simulink model "board_programmer"  (R2021b)
settings: Solver=FixedStepAuto  StartTime=0.0  StopTime=inf  RelTol=1e-3  EnableMultiTasking=on
values from neighbouring files (symbols this model uses):
  circ1 = monza    [board_data.m]
  serial_freq = 50    [board_data.m]
undefined symbols (not defined in the file or in its folder): CR, DiscIntNeverNeededParam, h, LF, pwm, slow, touch
libraries: simulink x19, dspstat3 x14, sharedschedule x12, arduinolib x5, simulink_extras x3, embeddedblockslib x2
settings Model: ExtModeTrigDuration=2  Creator=eduar  LastModifiedBy=ernesto
settings OptimizationCC: EnhancedBackFolding=on  PassReuseOutputArgsAs=Individual arguments  ZeroExternalMemoryAtStartup=off  ZeroInternalMemoryAtStartup=off  MaxStackSize=64  OptimizeBlockOrder=speed  DifferentSizesBufferReuse=on  OptimizationCustomize=off  EfficientTunableParamExpr=on
settings DebuggingCC: ParameterTunabilityLossMsg=error
settings HardwareCC: ProdBitPerPointer=32  ProdBitPerSizeT=32  ProdBitPerPtrDiffT=32  ProdLargestAtomicInteger=Long  ProdLargestAtomicFloat=Double  ProdWordSize=32  ProdHWDeviceType=ARM Compatible->ARM Cortex  UseEmbeddedCoderFeatures=off
settings SFSimCC: SimCustomHeaderCode="#include \"script\\callback.h\""  SimUserSources=script\callback.c  MATLABDynamicMemAlloc=off
settings RTWCC: Description=Embedded Coder  SystemTargetFile=ert.tlc  HardwareBoard=Arduino Due  TemplateMakefile=ert_default_tmf  RTWUseSimCustomCode=on  CustomHeaderCode="#include \"script\\callback.h\""  CustomSource=script\callback.c  Toolchain=Arduino ARM  BuildConfiguration=Faster Runs
settings CodeAppCC: ForceParamTrailComments=on  IgnoreCustomStorageClasses=off  OperatorAnnotations=on  SimulinkDataObjDesc=on  SFDataObjDesc=on  InsertBlockDesc=on
settings ERTTargetCC: SupportContinuousTime=on  SupportNonInlinedSFcns=on  SupportVariableSizeSignals=on  ExtModeTransport=3  ExtModeStaticAlloc=on  ExtModeStaticAllocSize=24576  ExtModeMexFile=ext_xcp  ExtModeIntrfLevel=Level2 - Open

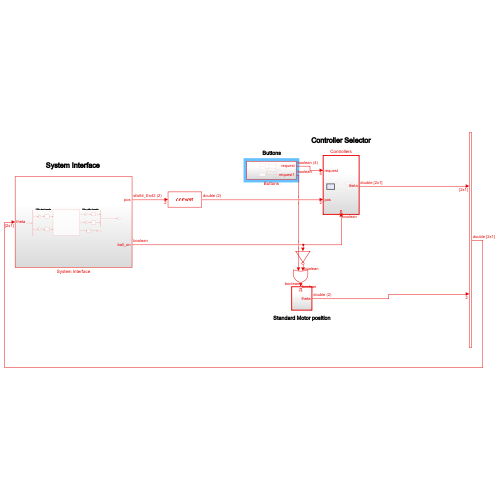
[thumbnail: Simulink's stored preview of the top-level diagram]
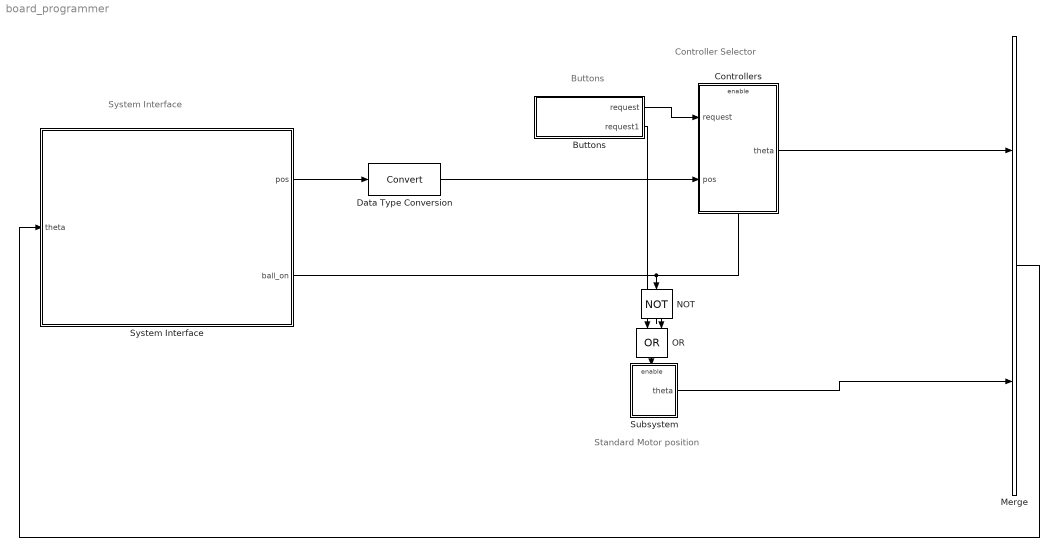
== system board_programmer ==
  note: Standard Motor position
  note: System Interface
  note: Controller Selector
  note: Buttons
  Buttons : Subsystem
  Controllers : Subsystem
  Data Type Conversion : DataTypeConversion
  Merge : Merge
  NOT : Logic  Operator=NOT  IconShape=distinctive  AllPortsSameDT=off  OutDataTypeStr=boolean
  OR : Logic  Operator=OR  IconShape=distinctive  AllPortsSameDT=off  OutDataTypeStr=boolean
  Subsystem : Subsystem
  System Interface : Subsystem
  wires:
  System Interface/1(pos) -> Data Type Conversion/1
  Controllers/1(theta) -> Merge/1
  Merge/1 -> System Interface/1(theta)
  Subsystem/1(theta) -> Merge/2
  System Interface/2(ball_on) -> NOT/1, Controllers/Enable
  Data Type Conversion/1 -> Controllers/2(pos)
  Buttons/1(request) -> Controllers/1(request)
  OR/1 -> Subsystem/Enable
  NOT/1 -> OR/2
  Buttons/2(request1) -> OR/1

== system board_programmer/Buttons ==
  AND : Logic  IconShape=distinctive  AllPortsSameDT=off  OutDataTypeStr=boolean
  Digital Input : arduinolib/Digital Input  pinNumber=7  mode=Input Pullup  Direction=input  SampleTime=0.02  blockPlatform=arduino
  Digital Input1 : arduinolib/Digital Input  pinNumber=53  mode=Input Pullup  Direction=input  SampleTime=0.02  blockPlatform=arduino
  Digital Input2 : arduinolib/Digital Input  pinNumber=51  mode=Input Pullup  Direction=input  SampleTime=0.02  blockPlatform=arduino
  Mux : Mux
  NOT{1..4} (4 alike) : Logic  Operator=NOT  IconShape=distinctive  AllPortsSameDT=off  OutDataTypeStr=boolean
  request : Outport
  request1 : Outport  Port=2
  wires:
  Digital Input1/1 -> AND/1, NOT2/1
  Digital Input2/1 -> AND/2, NOT3/1
  Digital Input/1 -> NOT1/1
  Mux/1 -> request/1
  NOT3/1 -> Mux/4
  AND/1 -> NOT4/1
  NOT4/1 -> request1/1, Mux/3
  NOT2/1 -> Mux/2
  NOT1/1 -> Mux/1

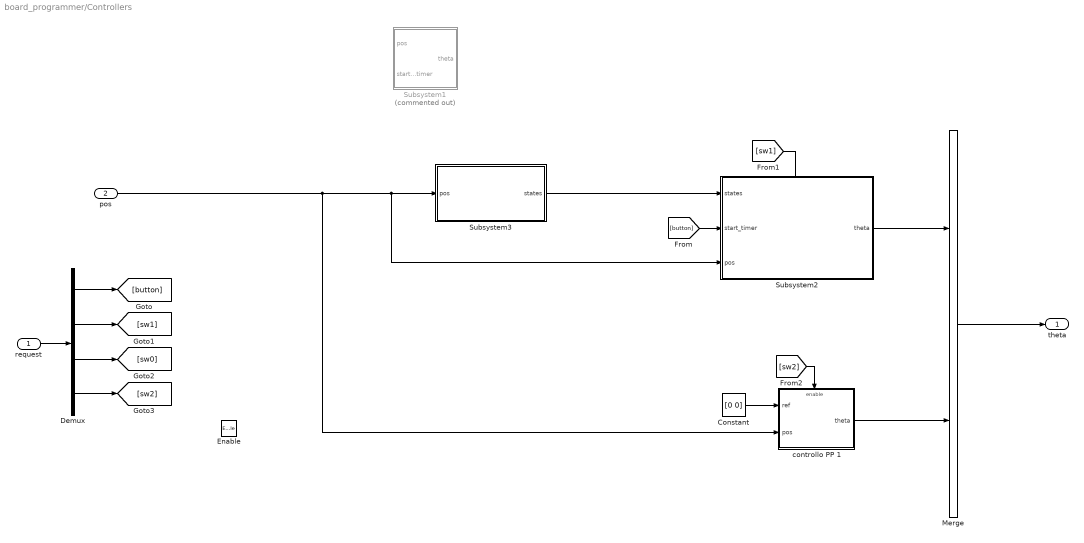
== system board_programmer/Controllers ==
  request : Inport
  pos : Inport  Port=2
  Enable : EnablePort
  Constant : Constant  Value=[0 0]
  Demux : Demux
  Merge : Merge
  Subsystem1 : Subsystem  Commented=on
  Subsystem2 : Subsystem
  Subsystem3 : Subsystem
  controllo PP 1 : Subsystem  SystemSampleTime=0.01
  theta : Outport
  wires:
  Subsystem3/1(states) -> Subsystem2/1(states)
  pos/1 -> controllo PP 1/2("pos "), Subsystem2/3(pos), Subsystem3/1(pos)
  request/1 -> Demux/1
  Demux/1 -> [button]
  Demux/2 -> [sw1]
  Demux/3 -> [sw0]
  Demux/4 -> [sw2]
  [button] -> Subsystem2/2(start_timer)
  [sw1] -> ?
  [sw2] -> controllo PP 1/Enable
  Constant/1 -> controllo PP 1/1("ref ")
  Subsystem2/1(theta) -> Merge/1
  Merge/1 -> theta/1
  controllo PP 1/1(theta) -> Merge/2

== system board_programmer/Subsystem ==
  Enable : EnablePort
  Constant1 : Constant  Value=[0 0]
  theta : Outport
  wires:
  Constant1/1 -> theta/1

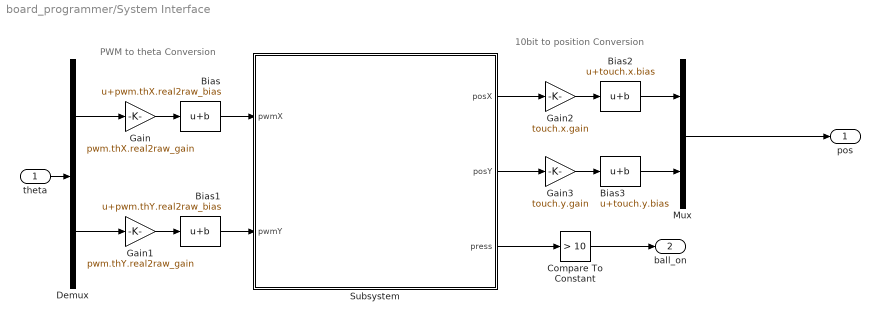
== system board_programmer/System Interface ==
  note: PWM to theta Conversion
  note: 10bit to position Conversion
  theta : Inport
  Bias : Bias  Bias=pwm.thX.real2raw_bias
  Bias1 : Bias  Bias=pwm.thY.real2raw_bias
  Bias2 : Bias  Bias=touch.x.bias
  Bias3 : Bias  Bias=touch.y.bias
  Compare To Constant : simulink/Logic and Bit Operations/Compare To Constant  relop=>  const=10  OutDataTypeStr=boolean
  Demux : Demux  Outputs=2
  Gain : Gain  Gain=pwm.thX.real2raw_gain
  Gain1 : Gain  Gain=pwm.thY.real2raw_gain
  Gain2 : Gain  Gain=touch.x.gain
  Gain3 : Gain  Gain=touch.y.gain
  Mux : Mux  Inputs=2
  Subsystem : Subsystem
  pos : Outport
  ball_on : Outport  Port=2
  wires:
  Subsystem/2(posY) -> Gain3/1
  Subsystem/1(posX) -> Gain2/1
  Bias2/1 -> Mux/1
  Gain/1 -> Bias/1
  Bias/1 -> Subsystem/1(pwmX)
  Demux/1 -> Gain/1
  Mux/1 -> pos/1
  Bias3/1 -> Mux/2
  Bias1/1 -> Subsystem/2(pwmY)
  theta/1 -> Demux/1
  Gain1/1 -> Bias1/1
  Demux/2 -> Gain1/1
  Gain2/1 -> Bias2/1
  Gain3/1 -> Bias3/1
  Subsystem/3(press) -> Compare To Constant/1
  Compare To Constant/1 -> ball_on/1

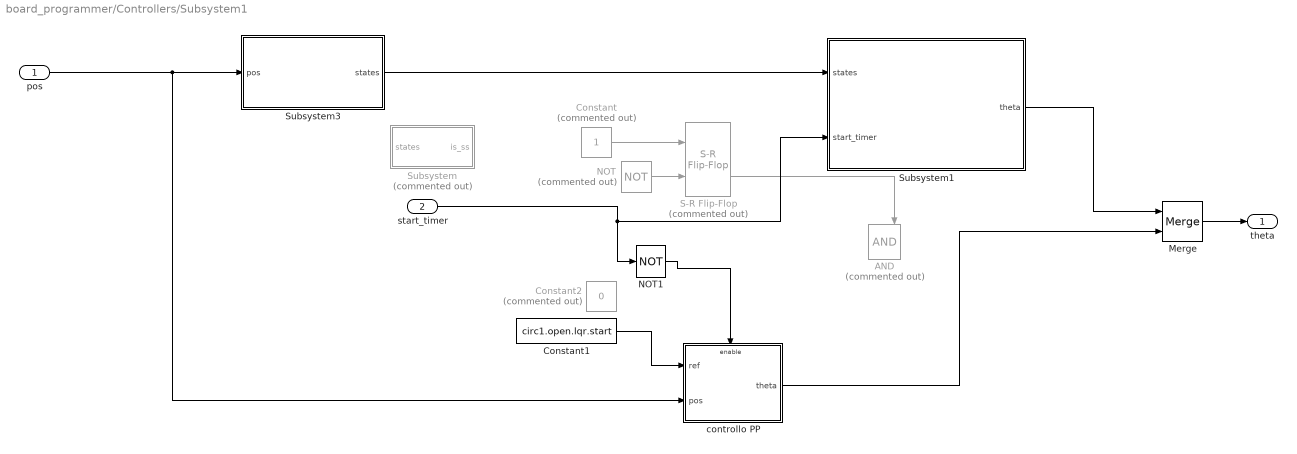
== system board_programmer/Controllers/Subsystem1 ==
  pos : Inport
  start_timer : Inport  Port=2
  AND : Logic  Commented=on  IconShape=distinctive  AllPortsSameDT=off  OutDataTypeStr=boolean
  Constant : Constant  Commented=on  OutDataTypeStr=boolean
  Constant1 : Constant  Value=circ1.open.lqr.start
  Constant2 : Constant  Commented=on  Value=0  OutDataTypeStr=boolean
  Merge : Merge
  NOT : Logic  Commented=on  Operator=NOT  IconShape=distinctive  AllPortsSameDT=off  OutDataTypeStr=boolean
  NOT1 : Logic  Operator=NOT  IconShape=distinctive  AllPortsSameDT=off  OutDataTypeStr=boolean
  S-R Flip-Flop : simulink_extras/Flip Flops/S-R Flip-Flop  Commented=on  initial_condition=0
  Subsystem : Subsystem  Commented=on
  Subsystem1 : Subsystem
  Subsystem3 : Subsystem
  "controllo PP " : Subsystem  SystemSampleTime=0.01
  theta : Outport
  wires:
  Subsystem3/1(states) -> Subsystem1/1(states)
  "controllo PP "/1(theta) -> Merge/2
  pos/1 -> "controllo PP "/2("pos "), Subsystem3/1(pos)
  Constant1/1 -> "controllo PP "/1("ref ")
  NOT/1 -> S-R Flip-Flop/2
  S-R Flip-Flop/2 -> AND/2
  Constant/1 -> S-R Flip-Flop/1
  start_timer/1 -> NOT1/1, Subsystem1/2(start_timer)
  NOT1/1 -> "controllo PP "/Enable
  Subsystem1/1(theta) -> Merge/1
  Merge/1 -> theta/1

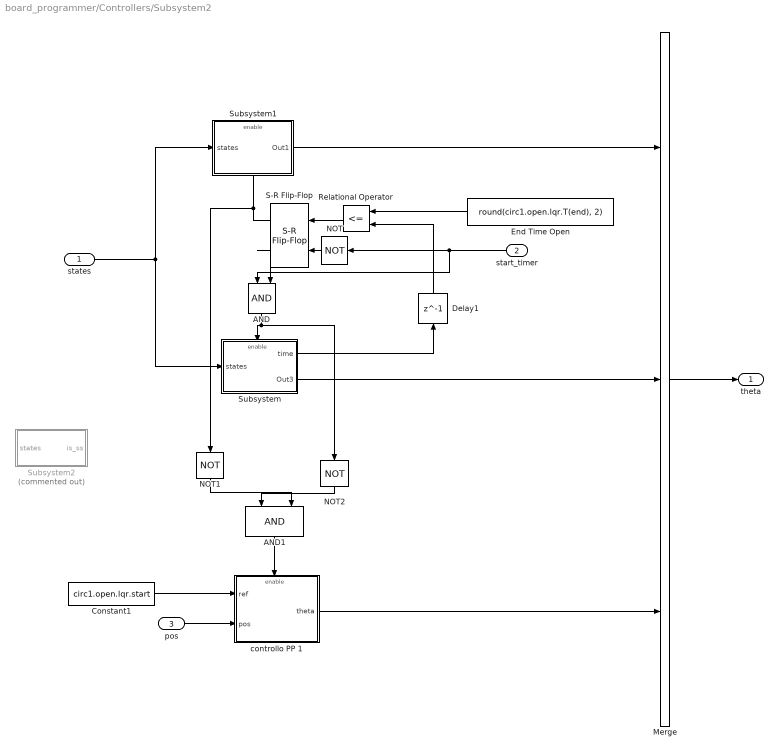
== system board_programmer/Controllers/Subsystem2 ==
  states : Inport
  start_timer : Inport  Port=2
  pos : Inport  Port=3
  AND : Logic  IconShape=distinctive  AllPortsSameDT=off  OutDataTypeStr=boolean
  AND1 : Logic  IconShape=distinctive  AllPortsSameDT=off  OutDataTypeStr=boolean
  Constant1 : Constant  Value=circ1.open.lqr.start
  Delay1 : Delay  DelayLength=1  InitialCondition=0
  End Time Open : Constant  Value=round(circ1.open.lqr.T(end), 2)
  Merge : Merge  Inputs=3
  NOT : Logic  Operator=NOT  IconShape=distinctive  AllPortsSameDT=off  OutDataTypeStr=boolean
  NOT1 : Logic  Operator=NOT  IconShape=distinctive  AllPortsSameDT=off  OutDataTypeStr=boolean
  NOT2 : Logic  Operator=NOT  IconShape=distinctive  AllPortsSameDT=off  OutDataTypeStr=boolean
  Relational Operator : RelationalOperator  Operator=<=  OutDataTypeStr=boolean  RndMeth=Simplest
  S-R Flip-Flop : simulink_extras/Flip Flops/S-R Flip-Flop  initial_condition=0
  Subsystem : Subsystem
  Subsystem1 : Subsystem
  Subsystem2 : Subsystem  Commented=on
  controllo PP 1 : Subsystem  SystemSampleTime=0.01
  theta : Outport
  wires:
  End Time Open/1 -> Relational Operator/1
  Relational Operator/1 -> S-R Flip-Flop/1
  S-R Flip-Flop/2 -> AND/1
  Merge/1 -> theta/1
  states/1 -> Subsystem1/1(states), Subsystem/1(states)
  Subsystem/1(time) -> Delay1/1
  Subsystem/2(Out3) -> Merge/2
  AND/1 -> NOT2/1, Subsystem/Enable
  Subsystem1/1(Out1) -> Merge/1
  S-R Flip-Flop/1 -> NOT1/1, Subsystem1/Enable
  Delay1/1 -> Relational Operator/2
  NOT/1 -> S-R Flip-Flop/2
  Constant1/1 -> controllo PP 1/1("ref ")
  controllo PP 1/1(theta) -> Merge/3
  pos/1 -> controllo PP 1/2("pos ")
  AND1/1 -> controllo PP 1/Enable
  NOT1/1 -> AND1/1
  NOT2/1 -> AND1/2
  start_timer/1 -> AND/2, NOT/1

== system board_programmer/Controllers/Subsystem3 ==
  pos : Inport
  Demux : Demux  Outputs=2
  Discrete Derivative : simulink/Discrete/Discrete Derivative  gainval=1.0  ICPrevScaledInput=0.0  OutMin=[]  OutMax=[]  OutDataType=fixdt(1, 16)  OutScaling=2^-10  DoSatur=off
  Discrete Derivative1 : simulink/Discrete/Discrete Derivative  gainval=1.0  ICPrevScaledInput=0.0  OutMin=[]  OutMax=[]  OutDataType=fixdt(1, 16)  OutScaling=2^-10  DoSatur=off
  Moving Average : dspstat3/Moving Average  Method=Sliding window  ForgettingFactorPort=off  SpecifyWindowLength=on  WindowLength=5  ForgettingFactor=0.9  SimulateUsing=Code generation
  Moving Average1 : dspstat3/Moving Average  Method=Sliding window  ForgettingFactorPort=off  SpecifyWindowLength=on  WindowLength=5  ForgettingFactor=0.9  SimulateUsing=Code generation
  Mux2 : Mux
  states : Outport
  wires:
  Discrete Derivative1/1 -> Moving Average1/1  "Xp [m/s]"
  Mux2/1 -> states/1
  Demux/2 -> Discrete Derivative1/1, Mux2/4
  Discrete Derivative/1 -> Moving Average/1  "Xp [m/s]"
  Demux/1 -> Mux2/2, Discrete Derivative/1
  pos/1 -> Demux/1
  Moving Average/1 -> Mux2/1
  Moving Average1/1 -> Mux2/3

== system board_programmer/Controllers/controllo PP 1 ==
  "ref " : Inport
  "pos " : Inport  Port=2
  Enable : EnablePort  StatesWhenEnabling=reset  ShowOutputPort=on
  Demux : Demux  Outputs=2
  Demux1 : Demux  Outputs=2
  Mux : Mux  Inputs=2
  PPX 1 : Subsystem
  PPX 2 : Subsystem
  Sum2 : Sum  Inputs=|-+
  Sum3 : Sum  Inputs=|-+
  theta : Outport
  wires:
  "ref "/1 -> Demux1/1
  "pos "/1 -> Demux/1
  Demux/1 -> PPX 1/1("pos "), Sum2/1
  Demux/2 -> PPX 2/1("pos "), Sum3/1
  Demux1/1 -> Sum2/2
  Demux1/2 -> Sum3/2
  Sum3/1 -> PPX 2/2(err)
  Sum2/1 -> PPX 1/2(err)
  PPX 2/1(V) -> Mux/2
  PPX 1/1(V) -> Mux/1
  Mux/1 -> theta/1
  Enable/1 -> PPX 2/3(tr), PPX 1/3(tr)

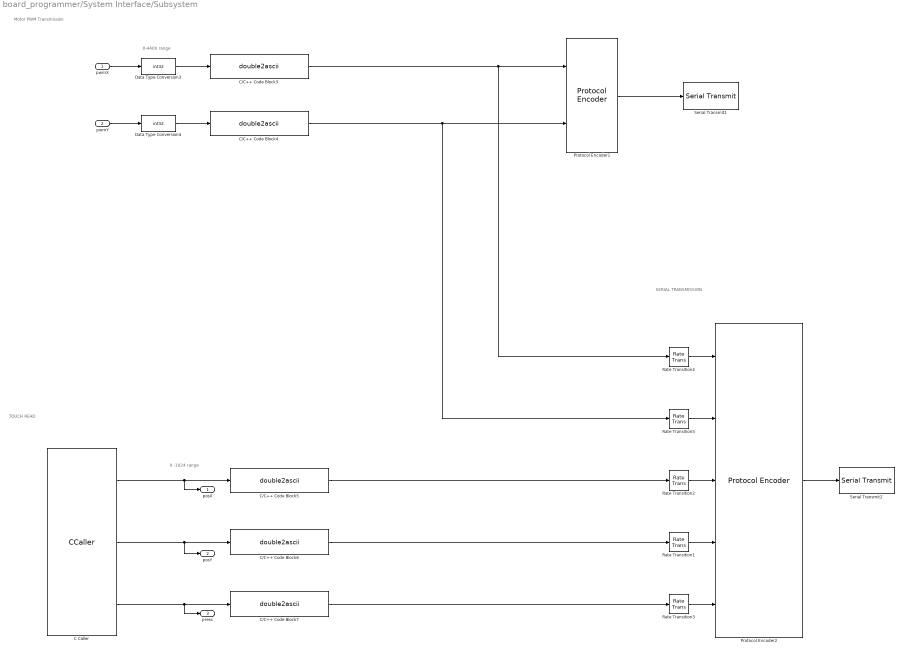
== system board_programmer/System Interface/Subsystem ==
  note: TOUCH READ
  note: Motor PWM Transmission
  note: 0 -1024 range
  note: 0-4400 range
  note: SERIAL TRANSMISSION
  pwmX : Inport
  pwmY : Inport  Port=2
  C Caller : CCaller  FunctionName=touchRead  PortSpecificationStruct="%)30     .    : 4   8    (     @         %    \"     ,    !     0         %  0 \"0    $    _    07)G3F%M90  4&]R=$YA;64 4V-O<&4     26YD97@     5'EP90      4VEZ90      27-';&]B86P   X    P    !@    @    $          4    (     0    $    !         !   0!X    #@   #     &    \"     0         !0    @    !     0    $         $  ! '@    .    .     8    (    !          %    \"     $    &     0         0    !@   $]U='!U=   #@   #@    &    \"     8         !0    @    !     0    $         \"0    @               X    X    !@    @    $          4    (     0    4    !         !     %    :6YT,S(    .    ,     8    (    !          %    \"     $    !     0         0  $ ,0    X    P    !@    @    ) @        4    (     0    $    !          (  0      #@   #     &    \"     0         !0    @    !     0    $         $  ! 'D    .    ,     8    (    !          %    \"     $    !     0         0  $ >0    X    X    !@    @    $          4    (     0    8    !         !     &    3W5T<'5T   .    .     8    (    !@         %    \"     $    !     0         )    \"            / _#@   #@    &    \"     0         !0    @    !    !0    $         $     4   !I;G0S,@    X    P    !@    @    $          4    (     0    $    !         !   0 Q    #@   #     &    \"     D\"        !0    @    !     0    $          @ !       .    .     8    (    !          %    \"     $    %     0         0    !0   '!R97-S    #@   #@    &    \"     0         !0    @    !    !0    $         $     4   !P<F5S<P    X    X    !@    @    $          4    (     0    8    !         !     &    3W5T<'5T   .    .     8    (    !@         %    \"     $    !     0         )    \"             ! #@   #@    &    \"     0         !0    @    !    !0    $         $     4   !I;G0S,@    X    P    !@    @    $          4    (     0    $    !         !   0 Q    #@   #     &    \"     D\"        !0    @    !     0    $          @ !"
  C/C++ Code Block3 : S-Function  FunctionName=double2ascii  SFunctionModules=double2ascii_wrapper  SFunctionDeploymentMode=off  EnableBusSupport=off  mask(S-Function Builder){}
      mask help: Simulink:masks:SFunctionBuilder_MD
      mask init:
      | val = [[.9  0.75 0.75 1 1 .9 .9 1]',[1 1 0.75 0.75 .9 .9 1 .9]'];try , sys = get_param(gcb,'SfunBuilderFcnName');if isempty(sys), sys = get_param(gcb,'FunctionName'); end,catch, sys = get_param(gcb,'FunctionName'); end
      settings: CopyFcn=set_param(gcbh,'LinkStatus','none')  OpenFcn=sfunctionwizard(gcbh)
      mask Display: plot(val(:,1),val(:,2)),disp(sys),port_label('input',1,'double_input'),port_label('output',1,'array_output')
  C/C++ Code Block4 : S-Function  FunctionName=double2ascii  SFunctionModules=double2ascii_wrapper  SFunctionDeploymentMode=off  EnableBusSupport=off  mask(S-Function Builder){}
      mask help: Simulink:masks:SFunctionBuilder_MD
      mask init: same as board_programmer/System Interface/Subsystem/C/C++ Code Block3
      settings: CopyFcn=set_param(gcbh,'LinkStatus','none')  OpenFcn=sfunctionwizard(gcbh)
      mask Display: plot(val(:,1),val(:,2)),disp(sys),port_label('input',1,'double_input'),port_label('output',1,'array_output')
  C/C++ Code Block5 : S-Function  FunctionName=double2ascii  SFunctionModules=double2ascii_wrapper  SFunctionDeploymentMode=off  EnableBusSupport=off  mask(S-Function Builder){}
      mask help: Simulink:masks:SFunctionBuilder_MD
      mask init: same as board_programmer/System Interface/Subsystem/C/C++ Code Block3
      settings: CopyFcn=set_param(gcbh,'LinkStatus','none')  OpenFcn=sfunctionwizard(gcbh)
      mask Display: plot(val(:,1),val(:,2)),disp(sys),port_label('input',1,'double_input'),port_label('output',1,'array_output')
  C/C++ Code Block6 : S-Function  FunctionName=double2ascii  SFunctionModules=double2ascii_wrapper  SFunctionDeploymentMode=off  EnableBusSupport=off  mask(S-Function Builder){}
      mask help: Simulink:masks:SFunctionBuilder_MD
      mask init: same as board_programmer/System Interface/Subsystem/C/C++ Code Block3
      settings: CopyFcn=set_param(gcbh,'LinkStatus','none')  OpenFcn=sfunctionwizard(gcbh)
      mask Display: plot(val(:,1),val(:,2)),disp(sys),port_label('input',1,'double_input'),port_label('output',1,'array_output')
  C/C++ Code Block7 : S-Function  FunctionName=double2ascii  SFunctionModules=double2ascii_wrapper  SFunctionDeploymentMode=off  EnableBusSupport=off  mask(S-Function Builder){}
      mask help: Simulink:masks:SFunctionBuilder_MD
      mask init: same as board_programmer/System Interface/Subsystem/C/C++ Code Block3
      settings: CopyFcn=set_param(gcbh,'LinkStatus','none')  OpenFcn=sfunctionwizard(gcbh)
      mask Display: plot(val(:,1),val(:,2)),disp(sys),port_label('input',1,'double_input'),port_label('output',1,'array_output')
  Data Type Conversion3 : DataTypeConversion  OutDataTypeStr=int32  RndMeth=Round
  Data Type Conversion4 : DataTypeConversion  OutDataTypeStr=int32  RndMeth=Round
  Protocol Encoder1 : embeddedblockslib/Protocol Encoder  Header='@'  FieldTable={ 'motX', '4', 'uint8', 'Little endian'; 'motY ', '4', 'uint8', 'Little endian' }  IsChecksumRequired=off  ChecksumAlgorithm=XOR of bytes  ChecksumSize=[]  TerminatorOption=CR/LF ('\r\n')  CustomTerminatorVal=[]  Logo=ARDUINO
      settings: SourceProductBaseCode=ARDUINO,TIC2000
  Protocol Encoder2 : embeddedblockslib/Protocol Encoder  Header='@'  FieldTable={ 'pwmX', '4', 'uint8', 'Little endian'; 'pwmY', '4', 'uint8', 'Little endian'; 'x', '4', 'uint8', 'Little endian'; 'y', '4', 'uint8', 'Little endian'; 'press', '4', 'uint8', 'Little endian' }  IsChecksumRequired=off  ChecksumAlgorithm=XOR of bytes  ChecksumSize=[]  TerminatorOption=CR/LF ('\r\n')  CustomTerminatorVal=[]  Logo=ARDUINO
      settings: SourceProductBaseCode=ARDUINO,TIC2000
  Rate Transition{1..5} (5 alike) : RateTransition  Integrity=off  OutPortSampleTime=1/serial_freq
  Serial Transmit1 : arduinolib/Serial Transmit  portNumber=3  sendmode=write  sendformat=Decimal  floatprecision=2  blockPlatform=arduino
  Serial Transmit2 : arduinolib/Serial Transmit  portNumber=0  sendmode=write  sendformat=Decimal  floatprecision=2  blockPlatform=arduino
  posX : Outport
  posY : Outport  Port=2
  press : Outport  Port=3
  wires:
  C Caller/2 -> posY/1, C/C++ Code Block6/1
  C/C++ Code Block3/1 -> Rate Transition4/1, Protocol Encoder1/1
  C/C++ Code Block4/1 -> Rate Transition5/1, Protocol Encoder1/2
  C Caller/3 -> press/1, C/C++ Code Block7/1
  C/C++ Code Block7/1 -> Rate Transition3/1
  C Caller/1 -> posX/1, C/C++ Code Block5/1
  C/C++ Code Block6/1 -> Rate Transition1/1
  C/C++ Code Block5/1 -> Rate Transition2/1
  Data Type Conversion4/1 -> C/C++ Code Block4/1
  Protocol Encoder1/1 -> Serial Transmit1/1
  pwmX/1 -> Data Type Conversion3/1
  Data Type Conversion3/1 -> C/C++ Code Block3/1
  pwmY/1 -> Data Type Conversion4/1
  Rate Transition3/1 -> Protocol Encoder2/5
  Rate Transition1/1 -> Protocol Encoder2/4
  Protocol Encoder2/1 -> Serial Transmit2/1
  Rate Transition4/1 -> Protocol Encoder2/1
  Rate Transition5/1 -> Protocol Encoder2/2
  Rate Transition2/1 -> Protocol Encoder2/3

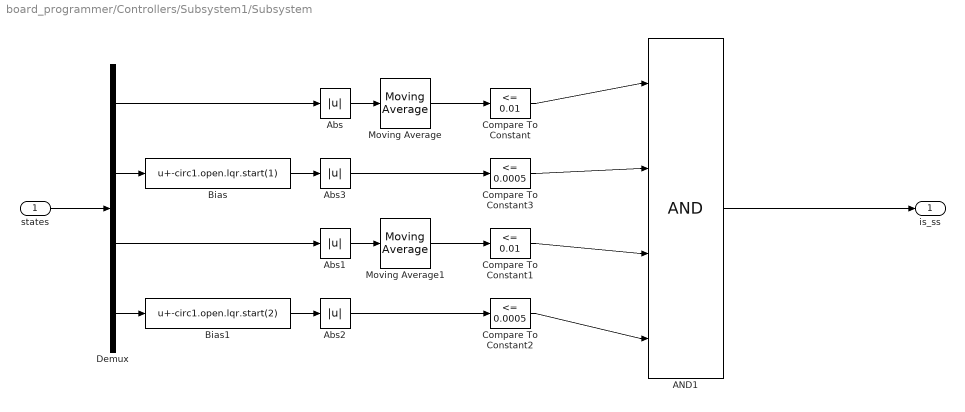
== system board_programmer/Controllers/Subsystem1/Subsystem ==
  states : Inport
  AND1 : Logic  Inputs=4  IconShape=distinctive  AllPortsSameDT=off  OutDataTypeStr=boolean
  Abs{,1..3} (4 alike) : Abs
  Bias : Bias  Bias=-circ1.open.lqr.start(1)
  Bias1 : Bias  Bias=-circ1.open.lqr.start(2)
  Compare To Constant : simulink/Logic and Bit Operations/Compare To Constant  relop=<=  const=0.01  OutDataTypeStr=boolean
  Compare To Constant1 : simulink/Logic and Bit Operations/Compare To Constant  relop=<=  const=0.01  OutDataTypeStr=boolean
  Compare To Constant2 : simulink/Logic and Bit Operations/Compare To Constant  relop=<=  const=0.0005  OutDataTypeStr=boolean
  Compare To Constant3 : simulink/Logic and Bit Operations/Compare To Constant  relop=<=  const=0.0005  OutDataTypeStr=boolean
  Demux : Demux
  Moving Average : dspstat3/Moving Average  Method=Sliding window  ForgettingFactorPort=off  SpecifyWindowLength=on  WindowLength=50  ForgettingFactor=0.9  SimulateUsing=Code generation
  Moving Average1 : dspstat3/Moving Average  Method=Sliding window  ForgettingFactorPort=off  SpecifyWindowLength=on  WindowLength=50  ForgettingFactor=0.9  SimulateUsing=Code generation
  is_ss : Outport
  wires:
  Moving Average1/1 -> Compare To Constant1/1
  Abs1/1 -> Moving Average1/1
  Moving Average/1 -> Compare To Constant/1
  AND1/1 -> is_ss/1
  Abs/1 -> Moving Average/1
  Compare To Constant/1 -> AND1/1
  Demux/1 -> Abs/1
  Demux/3 -> Abs1/1
  Compare To Constant1/1 -> AND1/3
  Demux/2 -> Bias/1
  Demux/4 -> Bias1/1
  Bias1/1 -> Abs2/1
  Bias/1 -> Abs3/1
  Abs2/1 -> Compare To Constant2/1
  Abs3/1 -> Compare To Constant3/1
  Compare To Constant2/1 -> AND1/4
  Compare To Constant3/1 -> AND1/2
  states/1 -> Demux/1

== system board_programmer/Controllers/Subsystem1/Subsystem1 ==
  states : Inport
  start_timer : Inport  Port=2
  AND : Logic  IconShape=distinctive  AllPortsSameDT=off  OutDataTypeStr=boolean
  Delay1 : Delay  DelayLength=1  InitialCondition=0
  End Time Open : Constant  Value=round(circ1.open.lqr.T(end), 2)
  Merge : Merge
  NOT : Logic  Operator=NOT  IconShape=distinctive  AllPortsSameDT=off  OutDataTypeStr=boolean
  Relational Operator : RelationalOperator  Operator=<=  OutDataTypeStr=boolean  RndMeth=Simplest
  S-R Flip-Flop : simulink_extras/Flip Flops/S-R Flip-Flop  initial_condition=0
  Subsystem : Subsystem
  Subsystem1 : Subsystem
  theta : Outport
  wires:
  start_timer/1 -> NOT/1, AND/2
  End Time Open/1 -> Relational Operator/1
  Relational Operator/1 -> S-R Flip-Flop/1
  NOT/1 -> S-R Flip-Flop/2
  S-R Flip-Flop/2 -> AND/1
  Merge/1 -> theta/1
  states/1 -> Subsystem1/1(states), Subsystem/1(states)
  Subsystem/1(time) -> Delay1/1
  Subsystem/2(Out3) -> Merge/2
  AND/1 -> Subsystem/Enable
  Subsystem1/1(Out1) -> Merge/1
  S-R Flip-Flop/1 -> Subsystem1/Enable
  Delay1/1 -> Relational Operator/2

== system board_programmer/Controllers/Subsystem1/Subsystem3 ==
  pos : Inport
  Demux : Demux  Outputs=2
  Discrete Derivative : simulink/Discrete/Discrete Derivative  gainval=1.0  ICPrevScaledInput=0.0  OutMin=[]  OutMax=[]  OutDataType=fixdt(1, 16)  OutScaling=2^-10  DoSatur=off
  Discrete Derivative1 : simulink/Discrete/Discrete Derivative  gainval=1.0  ICPrevScaledInput=0.0  OutMin=[]  OutMax=[]  OutDataType=fixdt(1, 16)  OutScaling=2^-10  DoSatur=off
  Moving Average : dspstat3/Moving Average  Method=Sliding window  ForgettingFactorPort=off  SpecifyWindowLength=on  WindowLength=5  ForgettingFactor=0.9  SimulateUsing=Code generation
  Moving Average1 : dspstat3/Moving Average  Method=Sliding window  ForgettingFactorPort=off  SpecifyWindowLength=on  WindowLength=5  ForgettingFactor=0.9  SimulateUsing=Code generation
  Mux2 : Mux
  states : Outport
  wires:
  Discrete Derivative1/1 -> Moving Average1/1  "Xp [m/s]"
  Mux2/1 -> states/1
  Demux/2 -> Discrete Derivative1/1, Mux2/4
  Discrete Derivative/1 -> Moving Average/1  "Xp [m/s]"
  Demux/1 -> Mux2/2, Discrete Derivative/1
  pos/1 -> Demux/1
  Moving Average/1 -> Mux2/1
  Moving Average1/1 -> Mux2/3

== system board_programmer/Controllers/Subsystem1/controllo PP  ==
  "ref " : Inport
  "pos " : Inport  Port=2
  Enable : EnablePort  StatesWhenEnabling=reset  ShowOutputPort=on
  Demux : Demux  Outputs=2
  Demux1 : Demux  Outputs=2
  Mux : Mux  Inputs=2
  PPX 1 : Subsystem
  PPX 2 : Subsystem
  Sum2 : Sum  Inputs=|-+
  Sum3 : Sum  Inputs=|-+
  theta : Outport
  wires:
  "ref "/1 -> Demux1/1
  "pos "/1 -> Demux/1
  Demux/1 -> PPX 1/1("pos "), Sum2/1
  Demux/2 -> PPX 2/1("pos "), Sum3/1
  Demux1/1 -> Sum2/2
  Demux1/2 -> Sum3/2
  Sum3/1 -> PPX 2/2(err)
  Sum2/1 -> PPX 1/2(err)
  PPX 2/1(V) -> Mux/2
  PPX 1/1(V) -> Mux/1
  Mux/1 -> theta/1
  Enable/1 -> PPX 2/3(tr), PPX 1/3(tr)

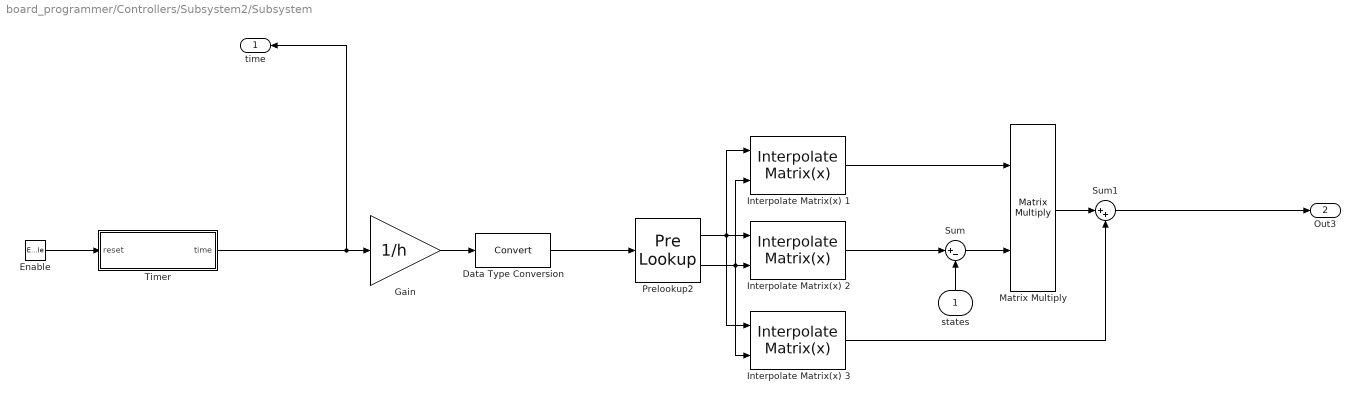
== system board_programmer/Controllers/Subsystem2/Subsystem ==
  states : Inport
  Enable : EnablePort  StatesWhenEnabling=reset  ShowOutputPort=on
  Data Type Conversion : DataTypeConversion
  Gain : Gain  Gain=1/h
  Interpolate Matrix(x) 1 : sharedschedule/Interpolate Matrix(x)   matrix=circ1.open.lqr.K  aMode=aMode
      settings: SourceProductBaseCode=AE,PW,DR,MT,UV,VE
  Interpolate Matrix(x) 2 : sharedschedule/Interpolate Matrix(x)   matrix=circ1.open.lqr.xk  aMode=aMode
      settings: SourceProductBaseCode=AE,PW,DR,MT,UV,VE
  Interpolate Matrix(x) 3 : sharedschedule/Interpolate Matrix(x)   matrix=circ1.open.lqr.uk  aMode=aMode
      settings: SourceProductBaseCode=AE,PW,DR,MT,UV,VE
  Matrix Multiply : Product  Multiplication=Matrix(*)
  Prelookup2 : PreLookup  BreakpointsData=([1:circ1.open.lqr.N])  IndexSearchMethod=Linear search  RemoveProtectionInput=on  BreakpointDataTypeStr=double  FractionDataTypeStr=double
  Sum : Sum  Inputs=|+-
  Sum1 : Sum  Inputs=|++
  "Timer " : Subsystem  TreatAsAtomicUnit=on
  time : Outport
  Out3 : Outport  Port=2
  wires:
  Interpolate Matrix(x) 2/1 -> Sum/1
  Data Type Conversion/1 -> Prelookup2/1
  Matrix Multiply/1 -> Sum1/1
  Interpolate Matrix(x) 3/1 -> Sum1/2
  Prelookup2/1 -> Interpolate Matrix(x) 1/1, Interpolate Matrix(x) 3/1, Interpolate Matrix(x) 2/1
  states/1 -> Sum/2
  Sum/1 -> Matrix Multiply/2
  "Timer "/1(time) -> time/1, Gain/1
  Gain/1 -> Data Type Conversion/1
  Prelookup2/2 -> Interpolate Matrix(x) 3/2, Interpolate Matrix(x) 1/2, Interpolate Matrix(x) 2/2
  Interpolate Matrix(x) 1/1 -> Matrix Multiply/1
  Sum1/1 -> Out3/1
  Enable/1 -> "Timer "/1(reset)

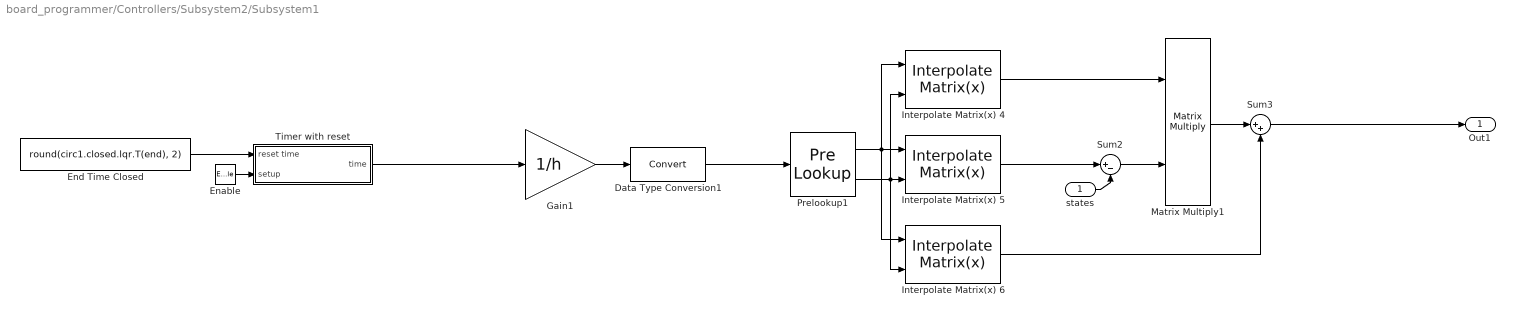
== system board_programmer/Controllers/Subsystem2/Subsystem1 ==
  states : Inport
  Enable : EnablePort  StatesWhenEnabling=reset  ShowOutputPort=on
  Data Type Conversion1 : DataTypeConversion
  End Time Closed : Constant  Value=round(circ1.closed.lqr.T(end), 2)
  Gain1 : Gain  Gain=1/h
  Interpolate Matrix(x) 4 : sharedschedule/Interpolate Matrix(x)   matrix=circ1.open.lqr.K  aMode=aMode
      settings: SourceProductBaseCode=AE,PW,DR,MT,UV,VE
  Interpolate Matrix(x) 5 : sharedschedule/Interpolate Matrix(x)   matrix=circ1.open.lqr.xk  aMode=aMode
      settings: SourceProductBaseCode=AE,PW,DR,MT,UV,VE
  Interpolate Matrix(x) 6 : sharedschedule/Interpolate Matrix(x)   matrix=circ1.open.lqr.uk  aMode=aMode
      settings: SourceProductBaseCode=AE,PW,DR,MT,UV,VE
  Matrix Multiply1 : Product  Multiplication=Matrix(*)
  Prelookup1 : PreLookup  BreakpointsData=([1:circ1.open.lqr.N])  IndexSearchMethod=Linear search  RemoveProtectionInput=on  BreakpointDataTypeStr=double  FractionDataTypeStr=double
  Sum2 : Sum  Inputs=|+-
  Sum3 : Sum  Inputs=|++
  Timer with reset : Subsystem  TreatAsAtomicUnit=on
  Out1 : Outport
  wires:
  Prelookup1/2 -> Interpolate Matrix(x) 6/2, Interpolate Matrix(x) 4/2, Interpolate Matrix(x) 5/2
  Prelookup1/1 -> Interpolate Matrix(x) 4/1, Interpolate Matrix(x) 6/1, Interpolate Matrix(x) 5/1
  Data Type Conversion1/1 -> Prelookup1/1
  Sum2/1 -> Matrix Multiply1/2
  Interpolate Matrix(x) 6/1 -> Sum3/2
  Gain1/1 -> Data Type Conversion1/1
  Interpolate Matrix(x) 5/1 -> Sum2/1
  Matrix Multiply1/1 -> Sum3/1
  End Time Closed/1 -> Timer with reset/1(reset time)
  Interpolate Matrix(x) 4/1 -> Matrix Multiply1/1
  Timer with reset/1(time) -> Gain1/1
  Sum3/1 -> Out1/1
  states/1 -> Sum2/2
  Enable/1 -> Timer with reset/2(setup)

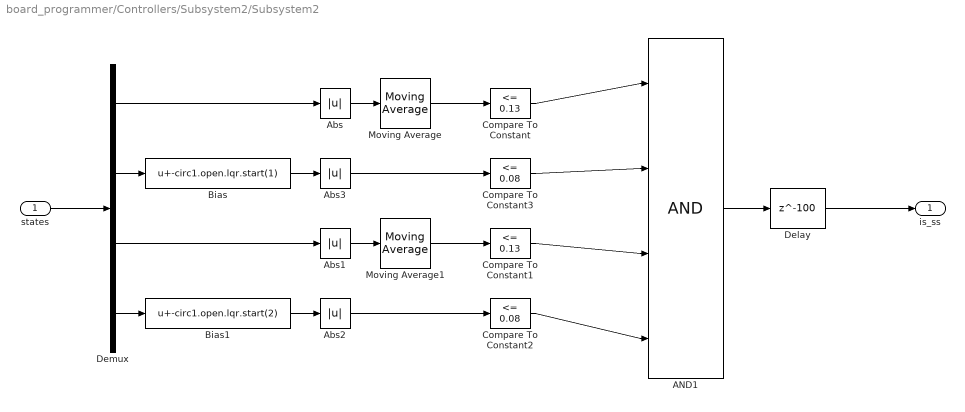
== system board_programmer/Controllers/Subsystem2/Subsystem2 ==
  states : Inport
  AND1 : Logic  Inputs=4  IconShape=distinctive  AllPortsSameDT=off  OutDataTypeStr=boolean
  Abs{,1..3} (4 alike) : Abs
  Bias : Bias  Bias=-circ1.open.lqr.start(1)
  Bias1 : Bias  Bias=-circ1.open.lqr.start(2)
  Compare To Constant : simulink/Logic and Bit Operations/Compare To Constant  relop=<=  const=0.13  OutDataTypeStr=boolean
  Compare To Constant1 : simulink/Logic and Bit Operations/Compare To Constant  relop=<=  const=0.13  OutDataTypeStr=boolean
  Compare To Constant2 : simulink/Logic and Bit Operations/Compare To Constant  relop=<=  const=0.08  OutDataTypeStr=boolean
  Compare To Constant3 : simulink/Logic and Bit Operations/Compare To Constant  relop=<=  const=0.08  OutDataTypeStr=boolean
  Delay : Delay  DelayLength=100  InputProcessing=Columns as channels (frame based)
  Demux : Demux
  Moving Average : dspstat3/Moving Average  Method=Sliding window  ForgettingFactorPort=off  SpecifyWindowLength=on  WindowLength=50  ForgettingFactor=0.9  SimulateUsing=Code generation
  Moving Average1 : dspstat3/Moving Average  Method=Sliding window  ForgettingFactorPort=off  SpecifyWindowLength=on  WindowLength=50  ForgettingFactor=0.9  SimulateUsing=Code generation
  is_ss : Outport
  wires:
  Moving Average1/1 -> Compare To Constant1/1
  Abs1/1 -> Moving Average1/1
  Moving Average/1 -> Compare To Constant/1
  AND1/1 -> Delay/1
  Abs/1 -> Moving Average/1
  Compare To Constant/1 -> AND1/1
  Demux/1 -> Abs/1
  Demux/3 -> Abs1/1
  Compare To Constant1/1 -> AND1/3
  Demux/2 -> Bias/1
  Demux/4 -> Bias1/1
  Bias1/1 -> Abs2/1
  Bias/1 -> Abs3/1
  Abs2/1 -> Compare To Constant2/1
  Abs3/1 -> Compare To Constant3/1
  Compare To Constant2/1 -> AND1/4
  Compare To Constant3/1 -> AND1/2
  states/1 -> Demux/1
  Delay/1 -> is_ss/1

== system board_programmer/Controllers/Subsystem2/controllo PP 1 ==
  "ref " : Inport
  "pos " : Inport  Port=2
  Enable : EnablePort  StatesWhenEnabling=reset  ShowOutputPort=on
  Demux : Demux  Outputs=2
  Demux1 : Demux  Outputs=2
  Mux : Mux  Inputs=2
  PPX 1 : Subsystem
  PPX 2 : Subsystem
  Sum2 : Sum  Inputs=|-+
  Sum3 : Sum  Inputs=|-+
  theta : Outport
  wires:
  "ref "/1 -> Demux1/1
  "pos "/1 -> Demux/1
  Demux/1 -> PPX 1/1("pos "), Sum2/1
  Demux/2 -> PPX 2/1("pos "), Sum3/1
  Demux1/1 -> Sum2/2
  Demux1/2 -> Sum3/2
  Sum3/1 -> PPX 2/2(err)
  Sum2/1 -> PPX 1/2(err)
  PPX 2/1(V) -> Mux/2
  PPX 1/1(V) -> Mux/1
  Mux/1 -> theta/1
  Enable/1 -> PPX 2/3(tr), PPX 1/3(tr)

== system board_programmer/Controllers/controllo PP 1/PPX 1 ==
  note: theta_x
  note: x_vel
  "pos " : Inport
  err : Inport  Port=2
  tr : Inport  Port=3
  Delay : Delay  DelayLength=1  InitialCondition=0
  Discrete Derivative : simulink/Discrete/Discrete Derivative  gainval=1.0  ICPrevScaledInput=0.0  OutMin=[]  OutMax=[]  OutDataType=fixdt(1, 16)  OutScaling=2^-10  DoSatur=off
  Discrete-Time Integrator : DiscreteIntegrator  ExternalReset=rising  SampleTime=-1  ICPrevOutput=DiscIntNeverNeededParam  ICPrevScaledInput=DiscIntNeverNeededParam
  Moving Average : dspstat3/Moving Average  Method=Sliding window  ForgettingFactorPort=off  SpecifyWindowLength=on  WindowLength=10  ForgettingFactor=0.9  SimulateUsing=Code generation
  Mux1 : Mux  Inputs=3
  Sum1 : Sum  Inputs=+|+
  Unary Minus : UnaryMinus
  x integration gain : Gain  Gain=slow.Kxi  Multiplication=Matrix(K*u)
  x matrix gain : Gain  Gain=slow.Kx  Multiplication=Matrix(K*u)
  V : Outport
  wires:
  x matrix gain/1 -> Sum1/1
  Mux1/1 -> x matrix gain/1  "x_vector"
  x integration gain/1 -> Sum1/2
  err/1 -> Discrete-Time Integrator/1, Mux1/2  "x_pos"
  Discrete-Time Integrator/1 -> x integration gain/1  "int_x"
  "pos "/1 -> Discrete Derivative/1
  Delay/1 -> Mux1/3
  Sum1/1 -> Delay/1, V/1
  tr/1 -> Discrete-Time Integrator/2  "x_pos"
  Discrete Derivative/1 -> Unary Minus/1
  Unary Minus/1 -> Moving Average/1
  Moving Average/1 -> Mux1/1

== system board_programmer/Controllers/controllo PP 1/PPX 2 ==
  note: theta_x
  note: x_vel
  "pos " : Inport
  err : Inport  Port=2
  tr : Inport  Port=3
  Delay : Delay  DelayLength=1  InitialCondition=0
  Discrete Derivative : simulink/Discrete/Discrete Derivative  gainval=1.0  ICPrevScaledInput=0.0  OutMin=[]  OutMax=[]  OutDataType=fixdt(1, 16)  OutScaling=2^-10  DoSatur=off
  Discrete-Time Integrator : DiscreteIntegrator  ExternalReset=rising  SampleTime=-1  ICPrevOutput=DiscIntNeverNeededParam  ICPrevScaledInput=DiscIntNeverNeededParam
  Moving Average : dspstat3/Moving Average  Method=Sliding window  ForgettingFactorPort=off  SpecifyWindowLength=on  WindowLength=10  ForgettingFactor=0.9  SimulateUsing=Code generation
  Mux1 : Mux  Inputs=3
  Sum1 : Sum  Inputs=+|+
  Unary Minus : UnaryMinus
  x integration gain : Gain  Gain=slow.Kyi  Multiplication=Matrix(K*u)
  x matrix gain : Gain  Gain=slow.Ky  Multiplication=Matrix(K*u)
  V : Outport
  wires:
  x matrix gain/1 -> Sum1/1
  Mux1/1 -> x matrix gain/1  "x_vector"
  x integration gain/1 -> Sum1/2
  err/1 -> Discrete-Time Integrator/1, Mux1/2  "x_pos"
  Discrete-Time Integrator/1 -> x integration gain/1  "int_x"
  "pos "/1 -> Discrete Derivative/1
  Delay/1 -> Mux1/3
  Sum1/1 -> Delay/1, V/1
  tr/1 -> Discrete-Time Integrator/2  "x_pos"
  Discrete Derivative/1 -> Unary Minus/1
  Unary Minus/1 -> Moving Average/1
  Moving Average/1 -> Mux1/1

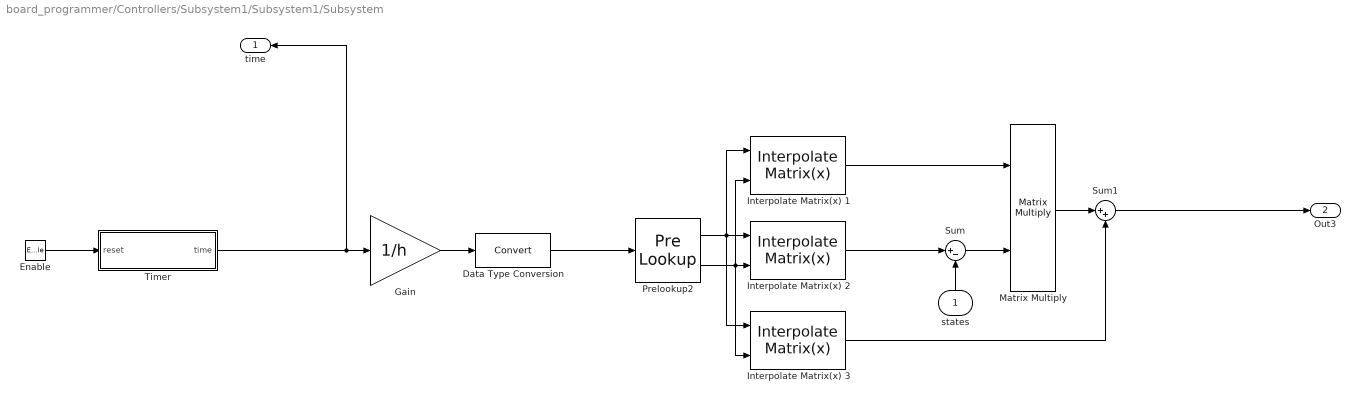
== system board_programmer/Controllers/Subsystem1/Subsystem1/Subsystem ==
  states : Inport
  Enable : EnablePort  StatesWhenEnabling=reset  ShowOutputPort=on
  Data Type Conversion : DataTypeConversion
  Gain : Gain  Gain=1/h
  Interpolate Matrix(x) 1 : sharedschedule/Interpolate Matrix(x)   matrix=circ1.open.lqr.K  aMode=aMode
      settings: SourceProductBaseCode=AE,PW,DR,MT,UV,VE
  Interpolate Matrix(x) 2 : sharedschedule/Interpolate Matrix(x)   matrix=circ1.open.lqr.xk  aMode=aMode
      settings: SourceProductBaseCode=AE,PW,DR,MT,UV,VE
  Interpolate Matrix(x) 3 : sharedschedule/Interpolate Matrix(x)   matrix=circ1.open.lqr.uk  aMode=aMode
      settings: SourceProductBaseCode=AE,PW,DR,MT,UV,VE
  Matrix Multiply : Product  Multiplication=Matrix(*)
  Prelookup2 : PreLookup  BreakpointsData=([1:circ1.open.lqr.N])  IndexSearchMethod=Linear search  RemoveProtectionInput=on  BreakpointDataTypeStr=double  FractionDataTypeStr=double
  Sum : Sum  Inputs=|+-
  Sum1 : Sum  Inputs=|++
  "Timer " : Subsystem  TreatAsAtomicUnit=on
  time : Outport
  Out3 : Outport  Port=2
  wires:
  Interpolate Matrix(x) 2/1 -> Sum/1
  Data Type Conversion/1 -> Prelookup2/1
  Matrix Multiply/1 -> Sum1/1
  Interpolate Matrix(x) 3/1 -> Sum1/2
  Prelookup2/1 -> Interpolate Matrix(x) 1/1, Interpolate Matrix(x) 3/1, Interpolate Matrix(x) 2/1
  states/1 -> Sum/2
  Sum/1 -> Matrix Multiply/2
  "Timer "/1(time) -> time/1, Gain/1
  Gain/1 -> Data Type Conversion/1
  Prelookup2/2 -> Interpolate Matrix(x) 3/2, Interpolate Matrix(x) 1/2, Interpolate Matrix(x) 2/2
  Interpolate Matrix(x) 1/1 -> Matrix Multiply/1
  Sum1/1 -> Out3/1
  Enable/1 -> "Timer "/1(reset)

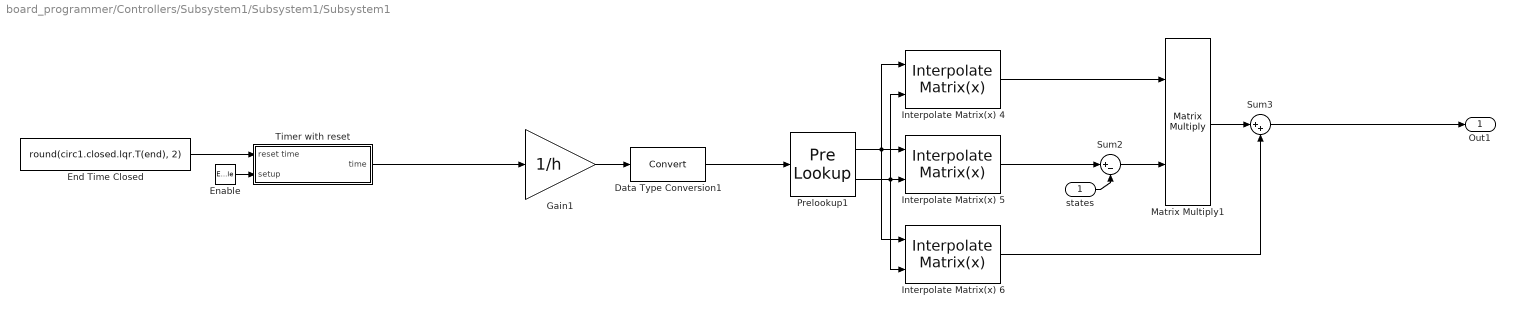
== system board_programmer/Controllers/Subsystem1/Subsystem1/Subsystem1 ==
  states : Inport
  Enable : EnablePort  StatesWhenEnabling=reset  ShowOutputPort=on
  Data Type Conversion1 : DataTypeConversion
  End Time Closed : Constant  Value=round(circ1.closed.lqr.T(end), 2)
  Gain1 : Gain  Gain=1/h
  Interpolate Matrix(x) 4 : sharedschedule/Interpolate Matrix(x)   matrix=circ1.open.lqr.K  aMode=aMode
      settings: SourceProductBaseCode=AE,PW,DR,MT,UV,VE
  Interpolate Matrix(x) 5 : sharedschedule/Interpolate Matrix(x)   matrix=circ1.open.lqr.xk  aMode=aMode
      settings: SourceProductBaseCode=AE,PW,DR,MT,UV,VE
  Interpolate Matrix(x) 6 : sharedschedule/Interpolate Matrix(x)   matrix=circ1.open.lqr.uk  aMode=aMode
      settings: SourceProductBaseCode=AE,PW,DR,MT,UV,VE
  Matrix Multiply1 : Product  Multiplication=Matrix(*)
  Prelookup1 : PreLookup  BreakpointsData=([1:circ1.open.lqr.N])  IndexSearchMethod=Linear search  RemoveProtectionInput=on  BreakpointDataTypeStr=double  FractionDataTypeStr=double
  Sum2 : Sum  Inputs=|+-
  Sum3 : Sum  Inputs=|++
  Timer with reset : Subsystem  TreatAsAtomicUnit=on
  Out1 : Outport
  wires:
  Prelookup1/2 -> Interpolate Matrix(x) 6/2, Interpolate Matrix(x) 4/2, Interpolate Matrix(x) 5/2
  Prelookup1/1 -> Interpolate Matrix(x) 4/1, Interpolate Matrix(x) 6/1, Interpolate Matrix(x) 5/1
  Data Type Conversion1/1 -> Prelookup1/1
  Sum2/1 -> Matrix Multiply1/2
  Interpolate Matrix(x) 6/1 -> Sum3/2
  Gain1/1 -> Data Type Conversion1/1
  Interpolate Matrix(x) 5/1 -> Sum2/1
  Matrix Multiply1/1 -> Sum3/1
  End Time Closed/1 -> Timer with reset/1(reset time)
  Interpolate Matrix(x) 4/1 -> Matrix Multiply1/1
  Timer with reset/1(time) -> Gain1/1
  Sum3/1 -> Out1/1
  states/1 -> Sum2/2
  Enable/1 -> Timer with reset/2(setup)

== system board_programmer/Controllers/Subsystem1/controllo PP /PPX 1 ==
  note: theta_x
  note: x_vel
  "pos " : Inport
  err : Inport  Port=2
  tr : Inport  Port=3
  Delay : Delay  DelayLength=1  InitialCondition=0
  Discrete Derivative : simulink/Discrete/Discrete Derivative  gainval=1.0  ICPrevScaledInput=0.0  OutMin=[]  OutMax=[]  OutDataType=fixdt(1, 16)  OutScaling=2^-10  DoSatur=off
  Discrete-Time Integrator : DiscreteIntegrator  ExternalReset=rising  SampleTime=-1  ICPrevOutput=DiscIntNeverNeededParam  ICPrevScaledInput=DiscIntNeverNeededParam
  Gain : Gain  Gain=0.15
  Moving Average : dspstat3/Moving Average  Method=Sliding window  ForgettingFactorPort=off  SpecifyWindowLength=on  WindowLength=20  ForgettingFactor=0.9  SimulateUsing=Code generation
  Mux1 : Mux  Inputs=3
  Sum1 : Sum  Inputs=+|+
  Unary Minus : UnaryMinus
  x integration gain : Gain  Gain=slow.Kxi  Multiplication=Matrix(K*u)
  x matrix gain : Gain  Gain=slow.Kx  Multiplication=Matrix(K*u)
  V : Outport
  wires:
  x matrix gain/1 -> Sum1/1
  Mux1/1 -> x matrix gain/1  "x_vector"
  x integration gain/1 -> Sum1/2
  err/1 -> Discrete-Time Integrator/1, Mux1/2  "x_pos"
  Discrete-Time Integrator/1 -> x integration gain/1  "int_x"
  Sum1/1 -> Gain/1
  "pos "/1 -> Discrete Derivative/1
  Delay/1 -> Mux1/3
  Gain/1 -> Delay/1, V/1
  tr/1 -> Discrete-Time Integrator/2  "x_pos"
  Discrete Derivative/1 -> Unary Minus/1
  Unary Minus/1 -> Moving Average/1
  Moving Average/1 -> Mux1/1

== system board_programmer/Controllers/Subsystem1/controllo PP /PPX 2 ==
  note: theta_x
  note: x_vel
  "pos " : Inport
  err : Inport  Port=2
  tr : Inport  Port=3
  Delay : Delay  DelayLength=1  InitialCondition=0
  Discrete Derivative : simulink/Discrete/Discrete Derivative  gainval=1.0  ICPrevScaledInput=0.0  OutMin=[]  OutMax=[]  OutDataType=fixdt(1, 16)  OutScaling=2^-10  DoSatur=off
  Discrete-Time Integrator : DiscreteIntegrator  ExternalReset=rising  SampleTime=-1  ICPrevOutput=DiscIntNeverNeededParam  ICPrevScaledInput=DiscIntNeverNeededParam
  Gain : Gain  Gain=0.15
  Moving Average : dspstat3/Moving Average  Method=Sliding window  ForgettingFactorPort=off  SpecifyWindowLength=on  WindowLength=10  ForgettingFactor=0.9  SimulateUsing=Code generation
  Mux1 : Mux  Inputs=3
  Sum1 : Sum  Inputs=+|+
  x integration gain : Gain  Gain=slow.Kyi  Multiplication=Matrix(K*u)
  x matrix gain : Gain  Gain=slow.Ky  Multiplication=Matrix(K*u)
  V : Outport
  wires:
  x matrix gain/1 -> Sum1/1
  Mux1/1 -> x matrix gain/1  "x_vector"
  x integration gain/1 -> Sum1/2
  err/1 -> Discrete-Time Integrator/1, Mux1/2  "x_pos"
  Discrete-Time Integrator/1 -> x integration gain/1  "int_x"
  Sum1/1 -> Gain/1
  "pos "/1 -> Discrete Derivative/1
  Delay/1 -> Mux1/3
  Gain/1 -> Delay/1, V/1
  tr/1 -> Discrete-Time Integrator/2  "x_pos"
  Discrete Derivative/1 -> Moving Average/1
  Moving Average/1 -> Mux1/1

== system board_programmer/Controllers/Subsystem2/Subsystem/Timer  ==
  reset : Inport
  Constant : Constant  SampleTime=-1
  Discrete-Time Integrator : DiscreteIntegrator  ExternalReset=either  SampleTime=-1  ICPrevOutput=DiscIntNeverNeededParam  ICPrevScaledInput=DiscIntNeverNeededParam
  time : Outport
  wires:
  Constant/1 -> Discrete-Time Integrator/1
  Discrete-Time Integrator/1 -> time/1
  reset/1 -> Discrete-Time Integrator/2

== system board_programmer/Controllers/Subsystem2/Subsystem1/Timer with reset ==
  reset time : Inport
  setup : Inport  Port=2
  AND : Logic  IconShape=distinctive  AllPortsSameDT=off  OutDataTypeStr=boolean
  Constant : Constant  SampleTime=-1
  Delay1 : Delay  DelayLength=1  InitialCondition=0
  Discrete-Time Integrator : DiscreteIntegrator  ExternalReset=either  SampleTime=-1  ICPrevOutput=DiscIntNeverNeededParam  ICPrevScaledInput=DiscIntNeverNeededParam
  Relational Operator : RelationalOperator  OutDataTypeStr=boolean  RndMeth=Simplest
  time : Outport
  wires:
  Constant/1 -> Discrete-Time Integrator/1
  Discrete-Time Integrator/1 -> Delay1/1, time/1
  AND/1 -> Discrete-Time Integrator/2
  setup/1 -> AND/1
  reset time/1 -> Relational Operator/2
  Delay1/1 -> Relational Operator/1
  Relational Operator/1 -> AND/2

== system board_programmer/Controllers/Subsystem2/controllo PP 1/PPX 1 ==
  note: theta_x
  note: x_vel
  "pos " : Inport
  err : Inport  Port=2
  tr : Inport  Port=3
  Delay : Delay  DelayLength=1  InitialCondition=0
  Discrete Derivative : simulink/Discrete/Discrete Derivative  gainval=1.0  ICPrevScaledInput=0.0  OutMin=[]  OutMax=[]  OutDataType=fixdt(1, 16)  OutScaling=2^-10  DoSatur=off
  Discrete-Time Integrator : DiscreteIntegrator  ExternalReset=rising  SampleTime=-1  ICPrevOutput=DiscIntNeverNeededParam  ICPrevScaledInput=DiscIntNeverNeededParam
  Moving Average : dspstat3/Moving Average  Method=Sliding window  ForgettingFactorPort=off  SpecifyWindowLength=on  WindowLength=10  ForgettingFactor=0.9  SimulateUsing=Code generation
  Mux1 : Mux  Inputs=3
  Sum1 : Sum  Inputs=+|+
  Unary Minus : UnaryMinus
  x integration gain : Gain  Gain=slow.Kxi  Multiplication=Matrix(K*u)
  x matrix gain : Gain  Gain=slow.Kx  Multiplication=Matrix(K*u)
  V : Outport
  wires:
  x matrix gain/1 -> Sum1/1
  Mux1/1 -> x matrix gain/1  "x_vector"
  x integration gain/1 -> Sum1/2
  err/1 -> Discrete-Time Integrator/1, Mux1/2  "x_pos"
  Discrete-Time Integrator/1 -> x integration gain/1  "int_x"
  "pos "/1 -> Discrete Derivative/1
  Delay/1 -> Mux1/3
  Sum1/1 -> Delay/1, V/1
  tr/1 -> Discrete-Time Integrator/2  "x_pos"
  Discrete Derivative/1 -> Unary Minus/1
  Unary Minus/1 -> Moving Average/1
  Moving Average/1 -> Mux1/1

== system board_programmer/Controllers/Subsystem2/controllo PP 1/PPX 2 ==
  note: theta_x
  note: x_vel
  "pos " : Inport
  err : Inport  Port=2
  tr : Inport  Port=3
  Delay : Delay  DelayLength=1  InitialCondition=0
  Discrete Derivative : simulink/Discrete/Discrete Derivative  gainval=1.0  ICPrevScaledInput=0.0  OutMin=[]  OutMax=[]  OutDataType=fixdt(1, 16)  OutScaling=2^-10  DoSatur=off
  Discrete-Time Integrator : DiscreteIntegrator  ExternalReset=rising  SampleTime=-1  ICPrevOutput=DiscIntNeverNeededParam  ICPrevScaledInput=DiscIntNeverNeededParam
  Moving Average : dspstat3/Moving Average  Method=Sliding window  ForgettingFactorPort=off  SpecifyWindowLength=on  WindowLength=10  ForgettingFactor=0.9  SimulateUsing=Code generation
  Mux1 : Mux  Inputs=3
  Sum1 : Sum  Inputs=+|+
  Unary Minus : UnaryMinus
  x integration gain : Gain  Gain=slow.Kyi  Multiplication=Matrix(K*u)
  x matrix gain : Gain  Gain=slow.Ky  Multiplication=Matrix(K*u)
  V : Outport
  wires:
  x matrix gain/1 -> Sum1/1
  Mux1/1 -> x matrix gain/1  "x_vector"
  x integration gain/1 -> Sum1/2
  err/1 -> Discrete-Time Integrator/1, Mux1/2  "x_pos"
  Discrete-Time Integrator/1 -> x integration gain/1  "int_x"
  "pos "/1 -> Discrete Derivative/1
  Delay/1 -> Mux1/3
  Sum1/1 -> Delay/1, V/1
  tr/1 -> Discrete-Time Integrator/2  "x_pos"
  Discrete Derivative/1 -> Unary Minus/1
  Unary Minus/1 -> Moving Average/1
  Moving Average/1 -> Mux1/1

== system board_programmer/Controllers/Subsystem1/Subsystem1/Subsystem/Timer  ==
  reset : Inport
  Constant : Constant  SampleTime=-1
  Discrete-Time Integrator : DiscreteIntegrator  ExternalReset=either  SampleTime=-1  ICPrevOutput=DiscIntNeverNeededParam  ICPrevScaledInput=DiscIntNeverNeededParam
  time : Outport
  wires:
  Constant/1 -> Discrete-Time Integrator/1
  Discrete-Time Integrator/1 -> time/1
  reset/1 -> Discrete-Time Integrator/2

== system board_programmer/Controllers/Subsystem1/Subsystem1/Subsystem1/Timer with reset ==
  reset time : Inport
  setup : Inport  Port=2
  AND : Logic  IconShape=distinctive  AllPortsSameDT=off  OutDataTypeStr=boolean
  Constant : Constant  SampleTime=-1
  Delay1 : Delay  DelayLength=1  InitialCondition=0
  Discrete-Time Integrator : DiscreteIntegrator  ExternalReset=either  SampleTime=-1  ICPrevOutput=DiscIntNeverNeededParam  ICPrevScaledInput=DiscIntNeverNeededParam
  Relational Operator : RelationalOperator  OutDataTypeStr=boolean  RndMeth=Simplest
  time : Outport
  wires:
  Constant/1 -> Discrete-Time Integrator/1
  Discrete-Time Integrator/1 -> Delay1/1, time/1
  AND/1 -> Discrete-Time Integrator/2
  setup/1 -> AND/1
  reset time/1 -> Relational Operator/2
  Delay1/1 -> Relational Operator/1
  Relational Operator/1 -> AND/2
